simulink model "Z_Transformation"  (R2020b)
settings: Solver=VariableStepAuto  StartTime=0.0  StopTime=10.0  RelTol=1e-3
settings Model: Creator=JAGRUTI SHINDE  LastModifiedBy=JAGRUTI SHINDE
settings DataIOCC: SaveOutput=off  SaveTime=off

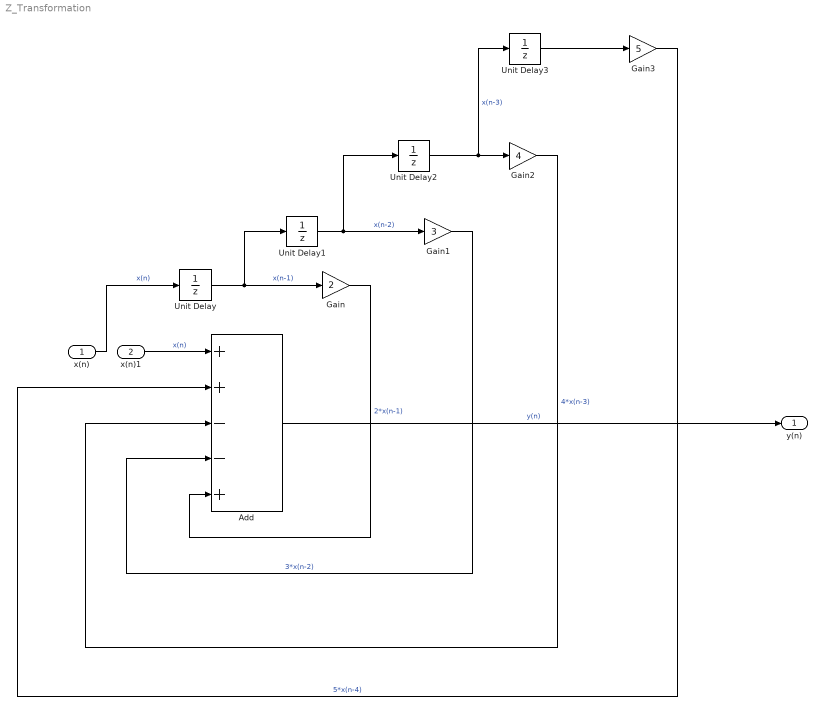
== system Z_Transformation ==
  x(n) : Inport  OutDataTypeStr=double  PortDimensions=1  SampleTime=[0,1]
  x(n)1 : Inport  Port=2  OutDataTypeStr=double  PortDimensions=1  SampleTime=[0,1]
  Add : Sum  Inputs=++--+
  Gain : Gain  Gain=2
  Gain1 : Gain  Gain=3
  Gain2 : Gain  Gain=4
  Gain3 : Gain  Gain=5
  Unit Delay{,1..3} (4 alike) : UnitDelay  SampleTime=-1  HasFrameUpgradeWarning=on
  y(n) : Outport  OutDataTypeStr=double  PortDimensions=1  SampleTime=[0,1]
  wires:
  Gain2/1 -> Add/3  "4*x(n-3)"
  Unit Delay2/1 -> Gain2/1, Unit Delay3/1  "x(n-3)"
  Gain3/1 -> Add/2  "5*x(n-4)"
  Gain/1 -> Add/5  "2*x(n-1)"
  Unit Delay/1 -> Gain/1, Unit Delay1/1  "x(n-1)"
  Gain1/1 -> Add/4  "3*x(n-2)"
  Unit Delay3/1 -> Gain3/1
  Unit Delay1/1 -> Gain1/1, Unit Delay2/1  "x(n-2)"
  x(n)/1 -> Unit Delay/1  "x(n)"
  Add/1 -> y(n)/1  "y(n)"
  x(n)1/1 -> Add/1  "x(n)"
